simulink model "model_FS_PSH_IEEE39"  (R2020b)
settings: Solver=ode3  StartTime=0.0  StopTime=300  FixedStep=Ts  RelTol=1e-3
PostLoadFcn:
  | IEEE39BusLineLength;
  | vNomHV = 345E3;fNom=60;load('Dynamicload.mat');
InitFcn:
  | IEEE39BusLineLength;
  | vNomHV = 345E3;fNom=60;load('Dynamicload.mat');
values from neighbouring files (symbols this model uses):
  Rp = 0.05    [IEEE39BusLineLength.m]
  t_sw_off = 220    [MAIN_FS_PSH_IEEE39.m]    (also in MAIN_T_PSH_IEEE39.m; MAIN_VS_PSH.m = 45)
  t_sw_on = 130    [MAIN_FS_PSH_IEEE39.m]    (also in MAIN_T_PSH_IEEE39.m; MAIN_VS_PSH.m = 35)
  TL_10_11_len = 14    [IEEE39BusLineLength.m]
  TL_10_13_len = 14    [IEEE39BusLineLength.m]
  TL_13_14_len = 32    [IEEE39BusLineLength.m]
  TL_14_15_len = 70    [IEEE39BusLineLength.m]
  TL_15_16_len = 31.5    [IEEE39BusLineLength.m]
  TL_16_17_len = 26    [IEEE39BusLineLength.m]
  TL_16_19_len = 61    [IEEE39BusLineLength.m]
  TL_16_21_len = 46    [IEEE39BusLineLength.m]
  TL_16_24_len = 15    [IEEE39BusLineLength.m]
  TL_17_18_len = 26    [IEEE39BusLineLength.m]
  TL_17_27_len = 59    [IEEE39BusLineLength.m]
  TL_1_2_len = 134    [IEEE39BusLineLength.m]
  TL_1_39_len = 105    [IEEE39BusLineLength.m]
  TL_21_22_len = 47    [IEEE39BusLineLength.m]
  TL_22_23_len = 33    [IEEE39BusLineLength.m]
  TL_24_23_len = 88    [IEEE39BusLineLength.m]
  TL_25_26_len = 101    [IEEE39BusLineLength.m]
  TL_26_27_len = 46.5    [IEEE39BusLineLength.m]
  TL_26_28_len = 151    [IEEE39BusLineLength.m]
  TL_26_29_len = 200    [IEEE39BusLineLength.m]
  TL_28_29_len = 48    [IEEE39BusLineLength.m]
  TL_2_25_len = 28    [IEEE39BusLineLength.m]
  TL_2_2_len = 49    [IEEE39BusLineLength.m]
  TL_3_18_len = 42    [IEEE39BusLineLength.m]
  TL_3_4_len = 53    [IEEE39BusLineLength.m]
  TL_4_14_len = 33    [IEEE39BusLineLength.m]
  TL_4_5_len = 32.5    [IEEE39BusLineLength.m]
  TL_5_6_len = 14    [IEEE39BusLineLength.m]
  TL_5_8_len = 32    [IEEE39BusLineLength.m]
  TL_6_11_len = 26.5    [IEEE39BusLineLength.m]
  TL_6_7_len = 25.5    [IEEE39BusLineLength.m]
  TL_7_8_len = 15    [IEEE39BusLineLength.m]
  TL_8_9_len = 93    [IEEE39BusLineLength.m]
  TL_9_39_len = 136    [IEEE39BusLineLength.m]
  Ts = 25e-6    (= 2.5e-05)    [MAIN_FS_PSH_IEEE39.m]    (also in MAIN_T_PSH_IEEE39.m; MAIN_VS_PSH.m = 1e-07)
undefined symbols (not defined in the file or in its folder): D1, Delta, FS_PSH, load15, load16, load18, load20, load21, load23, load24, load25, load26, load27, load28, load29, load3, load39, load4, load7, load8
libraries: powerlib x216, sps_avr x10, powerlib_meascontrol x5, pid_lib x1
(part 2 of 8)

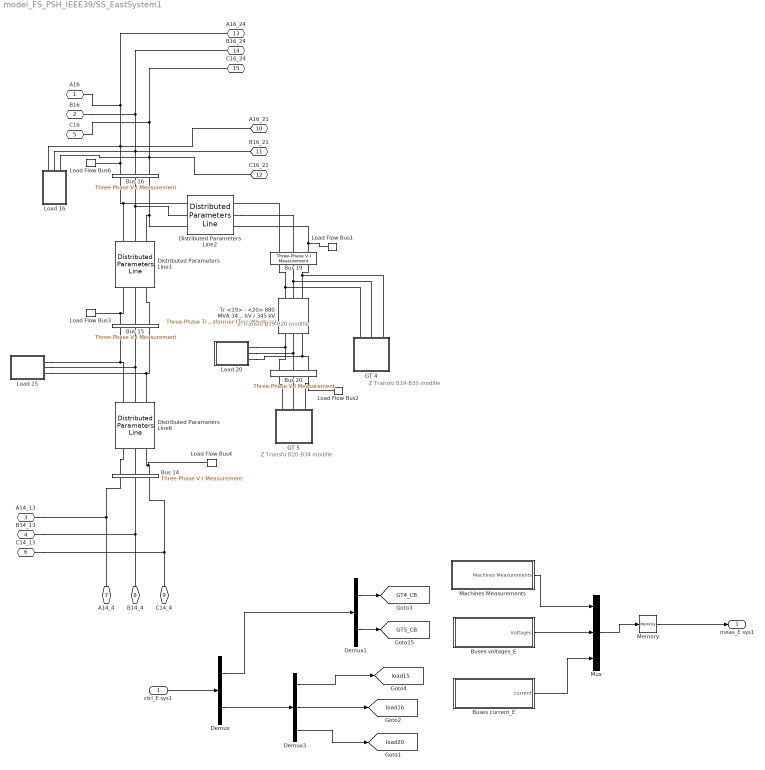
== system model_FS_PSH_IEEE39/SS_EastSystem1 ==
  note: Z Transfo B19-B20 modifie
  note: Z Transfo B20-B34 modifie
  note: Z Transfo B19-B33 modifie
  ctrl_E sys1 : Inport
  Bus 14 : powerlib/Measurements/Three-Phase V-I Measurement  VoltageMeasurement=phase-to-ground  SetLabelV=on  LabelV=V_bus_14  Vpu=off  VpuLL=off  CurrentMeasurement=yes  SetLabelI=on  LabelI=I_bus_14  Ipu=off  Pbase=100e6  Vbase=230e3  OutputType=Complex  PhasorSimulation=off  PSBequivalent=0
  Bus 15 : powerlib/Measurements/Three-Phase V-I Measurement  VoltageMeasurement=phase-to-ground  SetLabelV=on  LabelV=V_bus_15  Vpu=off  VpuLL=off  CurrentMeasurement=yes  SetLabelI=on  LabelI=I_bus_15  Ipu=off  Pbase=100e6  Vbase=230e3  OutputType=Complex  PhasorSimulation=off  PSBequivalent=0
  Bus 16 : powerlib/Measurements/Three-Phase V-I Measurement  VoltageMeasurement=phase-to-ground  SetLabelV=on  LabelV=V_bus_16  Vpu=off  VpuLL=off  CurrentMeasurement=yes  SetLabelI=on  LabelI=I_bus_16  Ipu=off  Pbase=100e6  Vbase=230e3  OutputType=Complex  PhasorSimulation=off  PSBequivalent=0
  Bus 19 : powerlib/Measurements/Three-Phase V-I Measurement  VoltageMeasurement=phase-to-ground  SetLabelV=on  LabelV=V_bus_19  Vpu=off  VpuLL=off  CurrentMeasurement=yes  SetLabelI=on  LabelI=I_bus_19  Ipu=off  Pbase=100e6  Vbase=230e3  OutputType=Complex  PhasorSimulation=off  PSBequivalent=0
  Bus 20 : powerlib/Measurements/Three-Phase V-I Measurement  VoltageMeasurement=phase-to-ground  SetLabelV=on  LabelV=V_bus_20  Vpu=off  VpuLL=off  CurrentMeasurement=yes  SetLabelI=on  LabelI=I_bus_20  Ipu=off  Pbase=100e6  Vbase=230e3  OutputType=Complex  PhasorSimulation=off  PSBequivalent=0
  Buses current_E : Subsystem
  Buses voltages_E : Subsystem
  Demux : Demux  Outputs=[2 6]
  Demux1 : Demux  Outputs=2
  Demux3 : Demux  Outputs=[2 2 2]
  Distributed Parameters Line1 : powerlib/Elements/Distributed Parameters Line  Phases=3  Length=TL_15_16_len  Frequency=fNom  Resistance=[1.071 4.285]/TL_15_16_len  Inductance=[0.03 0.089]/TL_15_16_len  Capacitance=[0.381e-6 0.173e-6]/TL_15_16_len  x1=[-0.000125 3.4902500343367e-08 265479.422569756 -48047.3717186245;-0.0001 3.46336269469464e-08 265014.796789079 -50547.2771775477;-7.5e-05 3.43616771915251e-08 264526.630861809 -53042.6927350425;-5e-05 3.40866752332531e-08 264014.968149667 -55533.3967338704;-2.5e-05 3.38086454993943e-08 263479.854101493 -58019.1679353007]  x2=[-0.000125 2.71337236080826e-08 262482.190210071 -41909.8217032638;-0.0001 2.68951060233545e-08 262075.54172196 -44381.7517104341;-7.5e-05 2.66540994597991e-08 261645.614168886 -46849.7394737977;-5e-05 2.6410725325013e-08 261192.4457395 -49313.5657724113;-2.5e-05 2.61650052368941e-08 260716.076686843 -51773.0117549771]  x3=[-0.000125 -7.17341676398892e-11 385.03003069748 -363.103493535617;-0.0001 -7.41140474713889e-11 381.590808633361 -366.716103516931;-7.5e-05 -7.64873440646573e-11 378.117691467223 -370.296139653542;-5e-05 -7.88538466097683e-11 374.610987701415 -373.843283945939;-2.5e-05 -8.12133449002827e-11 371.07100882164 -377.357221316256]  x4=[-0.000125 1.63179245843169e-10 1497.54093239525 81.2880799475028;-0.0001 1.64895753292141e-10 1498.24049440522 67.1707152946296;-7.5e-05 1.66597613746861e-10 1498.8069740315 53.0473841504362;-5e-05 1.68284676038245e-10 1499.2403209561 38.9193410308571;-2.5e-05 1.69956790311664e-10 1499.54049668663 24.7878408703722]  x5=0.000124084648526721  V1=ones(3,3)  V2=ones(3,3)  I1=ones(3,3)  I2=ones(3,3)  nHarmo=1  Measurements=None  Decoupling=off  VsMag0=0  VrMag0=0  VsAngle0=0  VrAngle0=0  IsMag0=0  IrMag0=0  IsAngle0=0  IrAngle0=0
  Distributed Parameters Line2 : powerlib/Elements/Distributed Parameters Line  Phases=3  Length=TL_16_19_len  Frequency=fNom  Resistance=[1.904 7.618]/TL_16_19_len  Inductance=[0.062 0.185]/TL_16_19_len  Capacitance=[0.677e-6 0.308e-6]/TL_16_19_len  x1=[-0.00025 3.61998957215348e-08 164457.7917293 -213872.689540181;-0.000225 3.59467568245282e-08 166466.150340024 -212313.23501404;-0.0002 3.56904249287326e-08 168459.722464751 -210734.921598748;-0.000175 3.54309228030293e-08 170438.331022878 -209137.88948923;-0.00015 3.51682734978974e-08 172401.800262951 -207522.280543111;-0.000125 3.4902500343367e-08 174349.955778281 -205888.23826812;-0.0001 3.46336269469464e-08 176282.624522429 -204235.907809339;-7.5e-05 3.43616771915251e-08 178199.634824584 -202565.435936314;-5e-05 3.40866752332531e-08 180100.816404805 -200876.971030016;-2.5e-05 3.38086454993943e-08 181986.000389152 -199170.66306966]  x2=[-0.00025 1.39140633367217e-07 179712.589064987 -204780.680260723;-0.000225 1.38613843536274e-07 181634.583034065 -203077.85776771;-0.0002 1.38074741222269e-07 183540.443169248 -201356.996725153;-0.000175 1.37523374311387e-07 185430.00018102 -199618.24998988;-0.00015 1.36959791779225e-07 187303.086228001 -197861.772007431;-0.000125 1.36384043686441e-07 189159.534931857 -196087.718798335;-0.0001 1.35796181174311e-07 190999.181392082 -194296.247944257;-7.5e-05 1.35196256460182e-07 192821.862200639 -192487.518573996;-5e-05 1.34584322832836e-07 194627.41545648 -190661.691349353;-2.5e-05 1.33960434647755e-07 196415.680779925 -188818.928450859]  x3=[-0.00025 6.09504380936159e-10 951.887942094555 -1339.93123171092;-0.000225 6.22475010302112e-10 964.473971369713 -1330.90044331579;-0.0002 6.35390347838437e-10 976.974330490048 -1321.75143664788;-0.000175 6.48249246330176e-10 989.387909101386 -1312.48502437487;-0.00015 6.61050563575614e-10 1001.7136045579 -1303.10202959308;-0.000125 6.73793162487735e-10 1013.95032202004 -1293.60328575435;-0.0001 6.86475911195223e-10 1026.09697455182 -1283.98963659204;-7.5e-05 6.99097683143007e-10 1038.15248321733 -1274.26193604604;-5e-05 7.11657357192321e-10 1050.11577717658 -1264.42104818698;-2.5e-05 7.24153817720295e-10 1061.98579378062 -1254.46784713941]  x4=[-0.00025 -3.80775285541496e-10 126.765412985895 -80.7754774079847;-0.000225 -3.9465237473206e-10 127.521063687958 -79.5772459689884;-0.0002 -4.0849440861678e-10 128.265387231805 -78.3719460188816;-0.000175 -4.22300157666171e-10 128.998317502315 -77.1596846193749;-0.00015 -4.36068395573776e-10 129.719789396383 -75.9405694505352;-0.000125 -4.49797899365095e-10 130.429738828704 -74.714708801221;-0.0001 -4.63487449506216e-10 131.128102737464 -73.4822115594631;-7.5e-05 -4.77135830012141e-10 131.814819089944 -72.243187202793;-5e-05 -4.90741828554797e-10 132.489826888025 -70.9977457885181;-2.5e-05 -5.04304236570722e-10 133.153066173613 -69.7459979439462]  x5=0.000238704838660635  V1=ones(3,3)  V2=ones(3,3)  I1=ones(3,3)  I2=ones(3,3)  nHarmo=1  Measurements=None  Decoupling=off  VsMag0=0  VrMag0=0  VsAngle0=0  VrAngle0=0  IsMag0=0  IrMag0=0  IsAngle0=0  IrAngle0=0
  Distributed Parameters Line6 : powerlib/Elements/Distributed Parameters Line  Phases=3  Length=TL_14_15_len  Frequency=fNom  Resistance=[2.142 8.57]/TL_14_15_len  Inductance=[0.069 0.206]/TL_14_15_len  Capacitance=[0.816e-6 0.371e-6]/TL_14_15_len  x1=[-0.0003 2.87345809506778e-08 0 0;-0.000275 2.85133357422329e-08 0 0;-0.00025 2.82895578144404e-08 264165.054992596 -29498.7341624213;-0.000225 2.80632670445498e-08 263875.302178294 -31987.0755016542;-0.0002 2.78344835330156e-08 263562.1104339 -34472.5755638885;-0.000175 2.76032276017123e-08 263225.507578914 -36955.0135726373;-0.00015 2.73695197921287e-08 262865.523512349 -39434.1690234031;-0.000125 2.71333808635439e-08 262482.190210071 -41909.8217032638;-0.0001 2.68948317911829e-08 262075.54172196 -44381.7517104341;-7.5e-05 2.66538937643535e-08 261645.614168886 -46849.7394737977;-5e-05 2.64105881845645e-08 261192.4457395 -49313.5657724113;-2.5e-05 2.61649366636243e-08 260716.076686843 -51773.0117549771]  x2=[-0.0003 6.24094556204278e-10 0 0;-0.000275 4.61999476276479e-10 0 0;-0.00025 2.99863358883869e-10 263159.120629807 -41326.7536874411;-0.000225 1.37700605893883e-10 262757.937699874 -43805.0887206173;-0.0002 -2.44743784601162e-11 262333.415090621 -46279.5327325279;-0.000175 -1.86647188858308e-10 261885.590510602 -48749.8659287483;-0.00015 -3.48803420173973e-10 261414.503738185 -51215.8688800003;-0.000125 -5.10928668753042e-10 260920.196618021 -53677.3225416431;-0.0001 -6.7300853369351e-10 260402.713057326 -56134.00827313;-7.5e-05 -8.35028618124614e-10 259862.099021983 -58585.7078574297;-5e-05 -9.96974530485636e-10 259298.402532457 -61032.203520409;-2.5e-05 -1.15883188580425e-09 258711.673659527 -63473.2779501774]  x3=[-0.0003 -7.80847688654747e-11 0 0;-0.000275 -8.16269036474497e-11 0 0;-0.00025 -8.51617878558679e-11 1355.39648204289 -135.7397363046;-0.000225 -8.86891075018747e-11 1354.05698540632 -148.507798254868;-0.0002 -9.22085492685438e-11 1352.59721359903 -161.262668883808;-0.000175 -9.57198005387079e-11 1351.01729628636 -174.003215230061;-0.00015 -9.92225494227265e-11 1349.31737380572 -186.728305604633;-0.000125 -1.02716484786191e-10 1347.49759715406 -199.436809691419;-0.0001 -1.06201296277559e-10 1345.55812797444 -212.127598647605;-7.5e-05 -1.09676674355726e-10 1343.49913854175 -224.799545203936;-5e-05 -1.13142310317515e-10 1341.32081174733 -237.451523764848;-2.5e-05 -1.16597896325101e-10 1339.02334108275 -250.082410508451]  x4=[-0.0003 1.19155637290744e-10 0 0;-0.000275 1.22199542792014e-10 0 0;-0.00025 1.25232593823324e-10 458.889537574224 -25.6157807215602;-0.000225 1.28254520971542e-10 458.627703746773 -29.9394798254312;-0.0002 1.31265055811628e-10 458.325131954845 -34.260519531591;-0.000175 1.34263930930469e-10 457.981849074614 -38.5785160203082;-0.00015 1.37250879950636e-10 457.597885598451 -42.8930857421677;-0.000125 1.40225637554049e-10 457.173275632212 -47.2038454521394;-0.0001 1.43187939505534e-10 456.70805689221 -51.5104122436206;-7.5e-05 1.46137522676307e-10 456.202270701863 -55.8124035824481;-5e-05 1.49074125067333e-10 455.655961988025 -60.1094373408764;-2.5e-05 1.51997485832609e-10 455.069179276995 -64.4011318315213]  x5=0.000276452527570286  V1=ones(3,3)  V2=ones(3,3)  I1=ones(3,3)  I2=ones(3,3)  nHarmo=1  Measurements=None  Decoupling=off  VsMag0=0  VrMag0=0  VsAngle0=0  VrAngle0=0  IsMag0=0  IrMag0=0  IsAngle0=0  IrAngle0=0
  GT 4 : Subsystem
  GT 5 : Subsystem
  Load 15 : Subsystem
  Load 16 : Subsystem
  Load 20 : Subsystem
  Load Flow Bus1 : powerlib/Measurements/Load Flow Bus  LConnTagsString=a  Phases=single  Connectors=on one side  ID=Bus-19  Vbase=345e+003  Vref=1  Vangle=0  VLF=1.019  VLFb=1  VLFc=1  angleLF=21.55  angleLFb=0  angleLFc=0
      settings: AttributesFormatString=%<ID>\n%<Vbase>V\n%<VLF>pu\n%<angleLF>deg.
  Load Flow Bus2 : powerlib/Measurements/Load Flow Bus  LConnTagsString=a  Phases=single  Connectors=on one side  ID=Bus-20  Vbase=345e+003  Vref=1  Vangle=0  VLF=0.9613  VLFb=1  VLFc=1  angleLF=-10.55  angleLFb=0  angleLFc=0
      settings: AttributesFormatString=%<ID>\n%<Vbase>V\n%<VLF>pu\n%<angleLF>deg.
  Load Flow Bus3 : powerlib/Measurements/Load Flow Bus  LConnTagsString=a  Phases=single  Connectors=on one side  ID=Bus-15  Vbase=345e+003  Vref=1  Vangle=0  VLF=0.996  VLFb=1  VLFc=1  angleLF=18.53  angleLFb=0  angleLFc=0
      settings: AttributesFormatString=%<ID>\n%<Vbase>V\n%<VLF>pu\n%<angleLF>deg.
  Load Flow Bus4 : powerlib/Measurements/Load Flow Bus  LConnTagsString=a  Phases=single  Connectors=on one side  ID=Bus-14  Vbase=345e+003  Vref=1  Vangle=0  VLF=1.001  VLFb=1  VLFc=1  angleLF=20.12  angleLFb=0  angleLFc=0
      settings: AttributesFormatString=%<ID>\n%<Vbase>V\n%<VLF>pu\n%<angleLF>deg.
  Load Flow Bus6 : powerlib/Measurements/Load Flow Bus  LConnTagsString=a  Phases=single  Connectors=on one side  ID=Bus-16  Vbase=345e+003  Vref=1  Vangle=0  VLF=1.007  VLFb=1  VLFc=1  angleLF=19.22  angleLFb=0  angleLFc=0
      settings: AttributesFormatString=%<ID>\n%<Vbase>V\n%<VLF>pu\n%<angleLF>deg.
  Machines Measurements : Subsystem
      mask Display: disp('Machines Measurements')
  Memory : Memory
  Mux : Mux  Inputs=3
  Tr <19> - <20> 880 MVA 345 kV / 345 kV : powerlib/Elements/Three-Phase Transformer (Two Windings)  Winding1Connection=Delta (D1)  Winding2Connection=Yg  CoreType=Three single-phase transformers  SetSaturation=off  Hysteresis=off  DataFile='hysteresis'  SetInitialFlux=off  Measurements=None  UNITS=pu  NominalPower=[ 880e6 fNom]  Winding1="[ 345e3 0.0007*880/100/2   0.0138*880/100/2 ]"  Winding2="[ 1.06*345e3 0.0007*880/100/2   0.0138*880/100/2 ]"  Rm=500  Lm=500  L0=0.5  Saturation="[ 0,0  ;  0.005,1.2  ;  1.0,1.4 ]"  InitialFluxes=[ 0.8 , -0.8 , 0.7 ]  BreakLoop=off  DiscreteSolver=Trapezoidal iterative  DataType=off  TransfoNumber=0
  A16 : PMIOPort  Side=Left
  B16 : PMIOPort  Port=2  Side=Left
  A14_13 : PMIOPort  Port=3  Side=Right
  B14_13 : PMIOPort  Port=4  Side=Right
  C16 : PMIOPort  Port=5  Side=Left
  C14_13 : PMIOPort  Port=6  Side=Right
  A14_4 : PMIOPort  Port=7  Side=Right
  B14_4 : PMIOPort  Port=8  Side=Right
  C14_4 : PMIOPort  Port=9  Side=Right
  A16_21 : PMIOPort  Port=10  Side=Left
  B16_21 : PMIOPort  Port=11  Side=Left
  C16_21 : PMIOPort  Port=12  Side=Left
  A16_24 : PMIOPort  Port=13  Side=Left
  B16_24 : PMIOPort  Port=14  Side=Left
  C16_24 : PMIOPort  Port=15  Side=Left
  meas_E sys1 : Outport
  tag scope: GT4_CB=global, GT5_CB=global, load15=global, load16=global, load20=global
  wires:
  Machines Measurements/1(Machines Measurements) -> Mux/1
  Mux/1 -> Memory/1
  Memory/1 -> meas_E sys1/1
  Buses voltages_E/1(Voltages) -> Mux/2
  Buses current_E/1(current) -> Mux/3
  ctrl_E sys1/1 -> Demux/1
  Demux/1 -> Demux1/1
  Demux1/2 -> [GT5_CB]
  Demux/2 -> Demux3/1
  Demux3/1 -> [load15]
  Demux3/2 -> [load16]
  Demux3/3 -> [load20]
  Demux1/1 -> [GT4_CB]
  connections:
  A14_4/RConn1 -- A14_13/RConn1 -- Bus 14/LConn1
  C14_4/RConn1 -- Bus 14/LConn3 -- C14_13/RConn1
  B14_4/RConn1 -- B14_13/RConn1 -- Bus 14/LConn2
  Tr <19> - <20> 880 MVA 345 kV / 345 kV/LConn3 -- Load 20/LConn3 -- Bus 20/RConn3
  Load 20/LConn2 -- Tr <19> - <20> 880 MVA 345 kV / 345 kV/LConn2 -- Bus 20/RConn2
  Load 20/LConn1 -- Tr <19> - <20> 880 MVA 345 kV / 345 kV/LConn1 -- Bus 20/RConn1
  GT 5/RConn3 -- Bus 20/LConn3 -- Load Flow Bus2/LConn1
  Bus 20/LConn2 -- GT 5/RConn2
  GT 5/RConn1 -- Bus 20/LConn1
  GT 4/RConn3 -- Tr <19> - <20> 880 MVA 345 kV / 345 kV/RConn3 -- Bus 19/LConn3
  GT 4/RConn2 -- Tr <19> - <20> 880 MVA 345 kV / 345 kV/RConn2 -- Bus 19/LConn2
  GT 4/RConn1 -- Tr <19> - <20> 880 MVA 345 kV / 345 kV/RConn1 -- Bus 19/LConn1
  C16/RConn1 -- C16_24/RConn1 -- Load 16/LConn3 -- Bus 16/RConn3 -- C16_21/RConn1
  B16/RConn1 -- B16_24/RConn1 -- Load 16/LConn2 -- B16_21/RConn1 -- Bus 16/RConn2
  Load Flow Bus6/LConn1 -- Bus 16/RConn1 -- Load 16/LConn1 -- A16_21/RConn1 -- A16_24/RConn1 -- A16/RConn1
  Bus 15/RConn3 -- Distributed Parameters Line1/RConn1
  Bus 15/RConn2 -- Distributed Parameters Line1/RConn2
  Bus 15/RConn1 -- Distributed Parameters Line1/RConn3 -- Load Flow Bus3/LConn1
  Bus 14/RConn3 -- Distributed Parameters Line6/RConn1 -- Load Flow Bus4/LConn1
  Bus 14/RConn2 -- Distributed Parameters Line6/RConn2
  Bus 14/RConn1 -- Distributed Parameters Line6/RConn3
  Bus 16/LConn1 -- Distributed Parameters Line2/LConn1 -- Distributed Parameters Line1/LConn3
  Bus 16/LConn2 -- Distributed Parameters Line1/LConn2 -- Distributed Parameters Line2/LConn2
  Bus 16/LConn3 -- Distributed Parameters Line2/LConn3 -- Distributed Parameters Line1/LConn1
  Load 15/LConn1 -- Distributed Parameters Line6/LConn3 -- Bus 15/LConn1
  Load 15/LConn2 -- Distributed Parameters Line6/LConn2 -- Bus 15/LConn2
  Bus 15/LConn3 -- Load 15/LConn3 -- Distributed Parameters Line6/LConn1
  Bus 19/RConn1 -- Distributed Parameters Line2/RConn1
  Distributed Parameters Line2/RConn2 -- Bus 19/RConn2
  Bus 19/RConn3 -- Distributed Parameters Line2/RConn3 -- Load Flow Bus1/LConn1

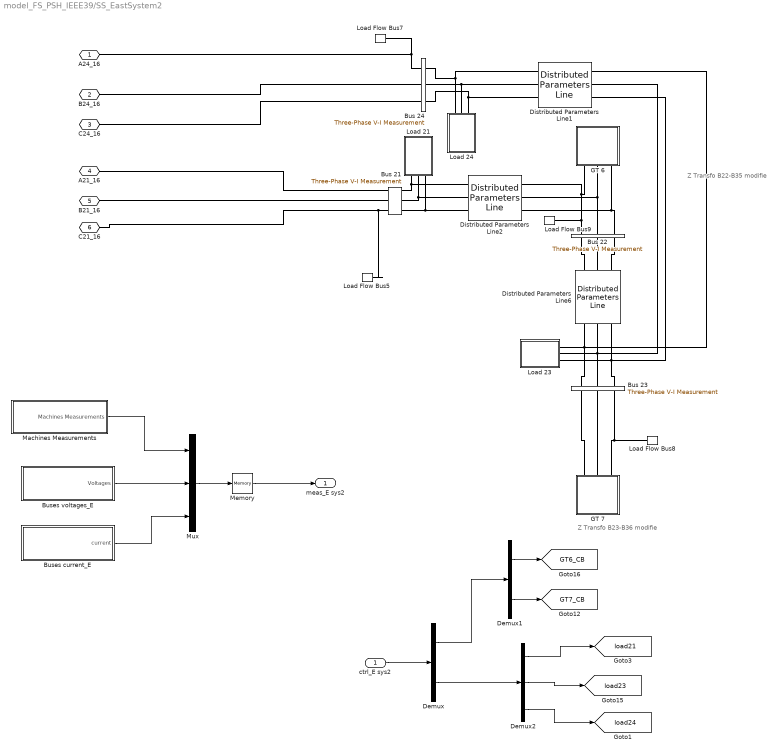
== system model_FS_PSH_IEEE39/SS_EastSystem2 ==
  note: Z Transfo B22-B35 modifie
  note: Z Transfo B23-B36 modifie
  ctrl_E sys2 : Inport
  Bus 21 : powerlib/Measurements/Three-Phase V-I Measurement  VoltageMeasurement=phase-to-ground  SetLabelV=on  LabelV=V_bus_21  Vpu=off  VpuLL=off  CurrentMeasurement=yes  SetLabelI=on  LabelI=I_bus_21  Ipu=off  Pbase=100e6  Vbase=230e3  OutputType=Complex  PhasorSimulation=off  PSBequivalent=0
  Bus 22 : powerlib/Measurements/Three-Phase V-I Measurement  VoltageMeasurement=phase-to-ground  SetLabelV=on  LabelV=V_bus_22  Vpu=off  VpuLL=off  CurrentMeasurement=yes  SetLabelI=on  LabelI=I_bus_22  Ipu=off  Pbase=100e6  Vbase=230e3  OutputType=Complex  PhasorSimulation=off  PSBequivalent=0
  Bus 23 : powerlib/Measurements/Three-Phase V-I Measurement  VoltageMeasurement=phase-to-ground  SetLabelV=on  LabelV=V_bus_23  Vpu=off  VpuLL=off  CurrentMeasurement=yes  SetLabelI=on  LabelI=I_bus_23  Ipu=off  Pbase=100e6  Vbase=230e3  OutputType=Complex  PhasorSimulation=off  PSBequivalent=0
  Bus 24 : powerlib/Measurements/Three-Phase V-I Measurement  VoltageMeasurement=phase-to-ground  SetLabelV=on  LabelV=V_bus_24  Vpu=off  VpuLL=off  CurrentMeasurement=yes  SetLabelI=on  LabelI=I_bus_24  Ipu=off  Pbase=100e6  Vbase=230e3  OutputType=Complex  PhasorSimulation=off  PSBequivalent=0
  Buses current_E : Subsystem
  Buses voltages_E : Subsystem
  Demux : Demux  Outputs=[2 6]
  Demux1 : Demux  Outputs=2
  Demux2 : Demux  Outputs=[2 2 2]
  Distributed Parameters Line1 : powerlib/Elements/Distributed Parameters Line  Phases=3  Length=TL_24_23_len  Frequency=fNom  Resistance=[2.619 10.474]/TL_24_23_len  Inductance=[0.111 0.332]/TL_24_23_len  Capacitance=[0.805e-6 0.365e-6]/TL_24_23_len  x1=[-0.00035 3.42625269720593e-08 156481.946701442 -221905.062565655;-0.000325 3.40524811440919e-08 158566.361734272 -220420.421229154;-0.0003 3.38394105778543e-08 160636.691986006 -218916.200876346;-0.000275 3.36233341995064e-08 162692.753557941 -217392.535120781;-0.00025 3.34042712022014e-08 164734.363818799 -215849.55930326;-0.000225 3.31822410443813e-08 166761.341420951 -214287.410479819;-0.0002 3.29572634480487e-08 168773.506316528 -212706.227409548;-0.000175 3.27293583970143e-08 170770.679773409 -211106.150542269;-0.00015 3.24985461351228e-08 172752.684391099 -209487.322006062;-0.000125 3.22648471644536e-08 174719.344116487 -207849.885594638;-0.0001 3.20282822435007e-08 176670.484259487 -206193.986754567;-7.5e-05 3.17888723853282e-08 178605.931508548 -204519.772572357;-5e-05 3.1546638855704e-08 180525.513946055 -202827.391761394;-2.5e-05 3.13016031712108e-08 182429.061063597 -201116.994648726]  x2=[-0.00035 3.41903240778697e-09 178835.393332096 -200303.621464305;-0.000325 3.50132440314296e-09 180715.229869132 -198609.266899253;-0.0003 3.58330539062045e-09 182579.014234537 -196897.270710737;-0.000275 3.66496808819412e-09 184426.580876208 -195167.784968156;-0.00025 3.74630524211098e-09 186257.765682592 -193420.963294434;-0.000225 3.82730962753472e-09 188072.405997267 -191656.960852374;-0.0002 3.90797404918746e-09 189870.340633388 -189875.93433087;-0.000175 3.98829134198885e-09 191651.409888005 -188078.041930998;-0.00015 4.06825437169255e-09 193415.455556247 -186263.443351955;-0.000125 4.14785603551989e-09 195162.32094538 -184432.299776879;-0.0001 4.22708926279084e-09 196891.850888718 -182584.773858532;-7.5e-05 4.30594701555202e-09 198603.891759412 -180721.029704847;-5e-05 4.38442228920186e-09 200298.291484092 -178841.232864356;-2.5e-05 4.46250811311279e-09 201974.899556377 -176945.550311484]  x3=[-0.00035 -2.27543163560437e-10 932.240108116287 -1117.42418668691;-0.000325 -2.29841235700864e-10 942.730009362682 -1108.58853334125;-0.0003 -2.32118892013772e-10 953.136171878686 -1099.65440875209;-0.000275 -2.34375930184556e-10 963.457671328774 -1090.62260650003;-0.00025 -2.36612149730036e-10 973.693590897686 -1081.49392884197;-0.000225 -2.38827352016262e-10 983.843021371861 -1072.26918663984;-0.0002 -2.41021340276158e-10 993.905061220198 -1062.94919928859;-0.000175 -2.43193919627001e-10 1003.87881667414 -1053.53479464339;-0.00015 -2.45344897087731e-10 1013.76340180705 -1044.02680894607;-0.000125 -2.47474081596093e-10 1023.55793861294 -1034.42608675092;-0.0001 -2.49581284025608e-10 1033.2615570844 -1024.73348084959;-7.5e-05 -2.51666317202371e-10 1042.87339528994 -1014.94985219537;-5e-05 -2.53728995921681e-10 1052.39259945052 -1005.07606982675;-2.5e-05 -2.55769136964486e-10 1061.81832401537 -995.113010790145]  x4=[-0.00035 2.6732583176681e-10 -97.905313643876 -64.336165130547;-0.000325 2.69508843962161e-10 -97.2946601678716 -65.2560331664969;-0.0003 2.71667916823665e-10 -96.6753644175837 -66.1701047842641;-0.000275 2.73802858569986e-10 -96.0474814024414 -67.0782987907221;-0.00025 2.75913479563252e-10 -95.4110668946449 -67.980534514828;-0.000225 2.77999592325904e-10 -94.7661774242104 -68.8767318147881;-0.0002 2.80061011557345e-10 -94.1128702739495 -69.7668110851762;-0.000175 2.82097554150398e-10 -93.4512034743808 -70.650693264005;-0.00015 2.84109039207575e-10 -92.7812357985753 -71.5282998397487;-0.000125 2.86095288057142e-10 -92.1030267569358 -72.3995528583168;-0.0001 2.88056124268993e-10 -91.4166365919107 -73.2643749299786;-7.5e-05 2.89991373670317e-10 -90.7221262726434 -74.1226892362371;-5e-05 2.91900864361072e-10 -90.0195574895561 -74.9744195366528;-2.5e-05 2.93784426729254e-10 -89.3089926488705 -75.8194901756157]  x5=0.000348109178276012  V1=ones(3,3)  V2=ones(3,3)  I1=ones(3,3)  I2=ones(3,3)  nHarmo=1  Measurements=None  Decoupling=off  VsMag0=0  VrMag0=0  VsAngle0=0  VrAngle0=0  IsMag0=0  IrMag0=0  IsAngle0=0  IrAngle0=0
  Distributed Parameters Line2 : powerlib/Elements/Distributed Parameters Line  Phases=3  Length=TL_21_22_len  Frequency=fNom  Resistance=[0.9522 3.809]/TL_21_22_len  Inductance=[0.044 0.133]/TL_21_22_len  Capacitance=[0.572e-6 0.26e-6]/TL_21_22_len  x1=[-0.0002 1.55933291358479e-08 0 0;-0.000175 1.53513573320371e-08 176314.466791581 -201742.801147765;-0.00015 1.51080219319049e-08 178207.978996054 -200072.140420211;-0.000125 1.48633445499086e-08 180085.661737416 -198383.708128307;-0.0001 1.46173469197081e-08 181947.348229028 -196677.654248373;-7.5e-05 1.43700508922352e-08 183792.873105134 -194954.130321979;-5e-05 1.41214784337529e-08 185622.072435541 -193213.289442485;-2.5e-05 1.38716516239044e-08 187434.783740189 -191455.286241445]  x2=[-0.0002 -6.22228426200295e-09 0 0;-0.000175 -6.41431381887781e-09 195027.702100886 -188379.951851512;-0.00015 -6.60577361931107e-09 196794.44318307 -186533.519372012;-0.000125 -6.79664665673621e-09 198543.703844925 -184670.517906765;-0.0001 -6.98691597670641e-09 200275.328707004 -182791.112938334;-7.5e-05 -7.17656467840051e-09 201989.163956376 -180895.471406336;-5e-05 -7.36557591612426e-09 203685.057360284 -178983.761692612;-2.5e-05 -7.55393290080664e-09 205362.858279669 -177056.153606272]  x3=[-0.0002 -1.1283053643262e-10 0 0;-0.000175 -1.17162459629033e-10 1478.83167899089 -1821.68219429991;-0.00015 -1.21483975778337e-10 1495.93467392415 -1807.66383326777;-0.000125 -1.2579470101848e-10 1512.90479129003 -1793.48490508187;-0.0001 -1.30094252445921e-10 1529.74052370459 -1779.1466691966;-7.5e-05 -1.34382248149642e-10 1546.44037572071 -1764.65039921695;-5e-05 -1.3865830724507e-10 1563.00286396099 -1749.99738278547;-2.5e-05 -1.42922049907912e-10 1579.42651724945 -1735.18892146778]  x4=[-0.0002 1.29050378263125e-10 0 0;-0.000175 1.32787243166402e-10 -185.385042295497 378.711216265608;-0.00015 1.36512313138951e-10 -188.946076045907 376.947210231573;-0.000125 1.40225257298519e-10 -192.490326513338 375.149721566777;-0.0001 1.43925745839937e-10 -196.017478876969 373.318909934559;-7.5e-05 1.47613450064417e-10 -199.527219834734 371.454937958194;-5e-05 1.51288042408746e-10 -203.019237631146 369.557971206448;-2.5e-05 1.54949196474386e-10 -206.493222084994 367.62817817888]  x5=0.000185956984273245  V1=ones(3,3)  V2=ones(3,3)  I1=ones(3,3)  I2=ones(3,3)  nHarmo=1  Measurements=None  Decoupling=off  VsMag0=0  VrMag0=0  VsAngle0=0  VrAngle0=0  IsMag0=0  IrMag0=0  IsAngle0=0  IrAngle0=0
  Distributed Parameters Line6 : powerlib/Elements/Distributed Parameters Line  Phases=3  Length=TL_22_23_len  Frequency=fNom  Resistance=[0.714 2.857]/TL_22_23_len  Inductance=[0.03 0.091]/TL_22_23_len  Capacitance=[0.411e-6 0.187e-6]/TL_22_23_len  x1=[-0.00015 5.54990165535425e-09 0 0;-0.000125 5.63270059276686e-09 195162.32094538 -184432.299776878;-0.0001 5.71499920114398e-09 196891.850888718 -182584.773858531;-7.5e-05 5.79679017024736e-09 198603.891759411 -180721.029704846;-5e-05 5.8780662349302e-09 200298.291484091 -178841.232864355;-2.5e-05 5.95882017578247e-09 201974.899556377 -176945.550311483]  x2=[-0.00015 -6.60577361931107e-09 0 0;-0.000125 -6.79664665673621e-09 198543.703844925 -184670.517906765;-0.0001 -6.98691597670641e-09 200275.328707004 -182791.112938334;-7.5e-05 -7.17656467840051e-09 201989.163956376 -180895.471406336;-5e-05 -7.36557591612426e-09 203685.057360284 -178983.761692612;-2.5e-05 -7.55393290080664e-09 205362.858279669 -177056.153606272]  x3=[-0.00015 8.17793319268742e-10 0 0;-0.000125 8.13923856051017e-10 704.478643864344 -995.209953136836;-0.0001 8.09982095410208e-10 713.826798542539 -988.526296882384;-7.5e-05 8.05968387476287e-10 723.11154699707 -981.754834006486;-5e-05 8.0188308877e-10 732.332064502892 -974.896165989626;-2.5e-05 7.97726562171201e-10 741.487532040328 -967.950902058355]  x4=[-0.00015 -8.19655310204693e-10 0 0;-0.000125 -8.15906171678577e-10 721.318718140451 -398.729130991085;-0.0001 -8.12084559648641e-10 725.044536945369 -391.913251517691;-7.5e-05 -8.08190813572562e-10 728.705953102236 -385.062560043215;-5e-05 -8.04225279315381e-10 732.302641382897 -378.177665085685;-2.5e-05 -8.00188309118781e-10 735.834282308703 -371.259178201281]  x5=0.000130449223838243  V1=ones(3,3)  V2=ones(3,3)  I1=ones(3,3)  I2=ones(3,3)  nHarmo=1  Measurements=None  Decoupling=off  VsMag0=0  VrMag0=0  VsAngle0=0  VrAngle0=0  IsMag0=0  IrMag0=0  IsAngle0=0  IrAngle0=0
  GT 6 : Subsystem
  GT 7 : Subsystem
  Load 21 : Subsystem
  Load 23 : Subsystem
  Load 24 : Subsystem
  Load Flow Bus5 : powerlib/Measurements/Load Flow Bus  LConnTagsString=a  Phases=single  Connectors=on one side  ID=Bus-21  Vbase=345e+003  Vref=1  Vangle=0  VLF=1.006  VLFb=1  VLFc=1  angleLF=20.56  angleLFb=0  angleLFc=0
      settings: AttributesFormatString=%<ID>\n%<Vbase>V\n%<VLF>pu\n%<angleLF>deg.
  Load Flow Bus7 : powerlib/Measurements/Load Flow Bus  LConnTagsString=a  Phases=single  Connectors=on one side  ID=Bus-24  Vbase=345e+003  Vref=1  Vangle=0  VLF=1.011  VLFb=1  VLFc=1  angleLF=19.08  angleLFb=0  angleLFc=0
      settings: AttributesFormatString=%<ID>\n%<Vbase>V\n%<VLF>pu\n%<angleLF>deg.
  Load Flow Bus8 : powerlib/Measurements/Load Flow Bus  LConnTagsString=a  Phases=single  Connectors=on one side  ID=Bus-23  Vbase=345e+003  Vref=1  Vangle=0  VLF=1.012  VLFb=1  VLFc=1  angleLF=23.42  angleLFb=0  angleLFc=0
      settings: AttributesFormatString=%<ID>\n%<Vbase>V\n%<VLF>pu\n%<angleLF>deg.
  Load Flow Bus9 : powerlib/Measurements/Load Flow Bus  LConnTagsString=a  Phases=single  Connectors=on one side  ID=Bus-22  Vbase=345e+003  Vref=1  Vangle=0  VLF=1.019  VLFb=1  VLFc=1  angleLF=23.66  angleLFb=0  angleLFc=0
      settings: AttributesFormatString=%<ID>\n%<Vbase>V\n%<VLF>pu\n%<angleLF>deg.
  Machines Measurements : Subsystem
      mask Display: disp('Machines Measurements')
  Memory : Memory
  Mux : Mux  Inputs=3
  A24_16 : PMIOPort  Side=Left
  B24_16 : PMIOPort  Port=2  Side=Left
  C24_16 : PMIOPort  Port=3  Side=Left
  A21_16 : PMIOPort  Port=4  Side=Left
  B21_16 : PMIOPort  Port=5  Side=Left
  C21_16 : PMIOPort  Port=6  Side=Left
  meas_E sys2 : Outport
  tag scope: GT6_CB=global, GT7_CB=global, load21=global, load23=global, load24=global
  wires:
  Machines Measurements/1(Machines Measurements) -> Mux/1
  Mux/1 -> Memory/1
  Memory/1 -> meas_E sys2/1
  Buses voltages_E/1(Voltages) -> Mux/2
  Buses current_E/1(current) -> Mux/3
  Demux/1 -> Demux1/1
  Demux/2 -> Demux2/1
  Demux1/2 -> [GT7_CB]
  Demux1/1 -> [GT6_CB]
  Demux2/1 -> [load21]
  Demux2/2 -> [load23]
  Demux2/3 -> [load24]
  ctrl_E sys2/1 -> Demux/1
  connections:
  Bus 24/RConn3 -- C24_16/RConn1
  Bus 24/RConn2 -- B24_16/RConn1
  Bus 24/RConn1 -- Load Flow Bus7/LConn1 -- A24_16/RConn1
  Load 23/LConn3 -- Distributed Parameters Line6/LConn3 -- Distributed Parameters Line1/RConn3 -- Bus 23/RConn3
  Load 23/LConn2 -- Distributed Parameters Line6/LConn2 -- Distributed Parameters Line1/RConn2 -- Bus 23/RConn2
  Load 23/LConn1 -- Distributed Parameters Line6/LConn1 -- Bus 23/RConn1 -- Distributed Parameters Line1/RConn1
  Load Flow Bus8/LConn1 -- GT 7/RConn3 -- Bus 23/LConn3
  Bus 22/RConn3 -- GT 6/RConn3 -- Distributed Parameters Line2/RConn3
  GT 6/RConn2 -- Bus 22/RConn2 -- Distributed Parameters Line2/RConn2
  Load Flow Bus9/LConn1 -- Distributed Parameters Line2/RConn1 -- GT 6/RConn1 -- Bus 22/RConn1
  Distributed Parameters Line6/RConn3 -- Bus 22/LConn3
  Distributed Parameters Line6/RConn2 -- Bus 22/LConn2
  Distributed Parameters Line6/RConn1 -- Bus 22/LConn1
  Bus 21/RConn1 -- Load 21/LConn1 -- Distributed Parameters Line2/LConn1
  Bus 21/RConn2 -- Load 21/LConn2 -- Distributed Parameters Line2/LConn2
  Bus 21/RConn3 -- Distributed Parameters Line2/LConn3 -- Load 21/LConn3
  C21_16/RConn1 -- Load Flow Bus5/LConn1 -- Bus 21/LConn3
  Load 24/LConn1 -- Distributed Parameters Line1/LConn1 -- Bus 24/LConn1
  Load 24/LConn2 -- Distributed Parameters Line1/LConn2 -- Bus 24/LConn2
  Bus 24/LConn3 -- Load 24/LConn3 -- Distributed Parameters Line1/LConn3
  Bus 21/LConn2 -- B21_16/RConn1
  A21_16/RConn1 -- Bus 21/LConn1
  GT 7/RConn1 -- Bus 23/LConn1
  GT 7/RConn2 -- Bus 23/LConn2
